simulink model "psm_mpc_bemf_ctrl"  (R2025b)
settings: Solver=ode23tb  StartTime=0.0  StopTime=simlength  FixedStep=tc  MaxStep=tc
values from neighbouring files (symbols this model uses):
  dead_time_INV = 3e-6    (= 3e-06)    [init_model.m]
  emf_fb_p = 0.2    [init_model.m]
  emf_fb_p_ccaller_1 = emf_fb_p    (= 0.2)    [init_model.m]
  emf_fb_p_ccaller_2 = emf_fb_p    (= 0.2)    [init_model.m]
  emf_p = emf_fb_p*4/10    (= 0.08)    [init_model.m]
  emf_p_ccaller_1 = emf_fb_p_ccaller_1*4/10    (= 0.08)    [init_model.m]
  emf_p_ccaller_2 = emf_fb_p_ccaller_2*4/10    (= 0.08)    [init_model.m]
  fPWM_INV = fPWM_AFE    (= 15000)    [init_model.m]
  g0_1Hz = fcut_1Hz_flt * ts_afe * 2*pi    (= 0.000418879020479)    [init_model.m]
  g1_1Hz = 1 - g0_1Hz    (= 0.99958112098)    [init_model.m]
  inv_m_scale = motorc_m_scale    [init_model.m]
  iq_lim = 1.4    [init_model.m]
  k_kalman = 0    [init_model.m]
  kg = Kobs(1)    [init_model.m]
  ki_w = 8    [init_model.m]
  kp_w = 2    [init_model.m]
  kw = Kobs(2)    [init_model.m]
  lim_down_align = -0.2    [init_model.m]
  lim_up_align = 0.2    [init_model.m]
  number_of_modules = 1    [init_model.m]
  omega_m_sim = omega_m_bez    [init_model.m]
  simlength = 2    [init_model.m]
  tc = ts_afe/100    (= 6.66666666667e-07)    [init_model.m]
  time_gain_afe_module_1 = 1.0    (= 1)    [init_model.m]
  time_gain_inv_module_2 = 1.0    (= 1)    [init_model.m]
  time_start_motor_control = 0.035    [init_model.m]
  ts_inv = 1/fPWM_INV    (= 6.66666666667e-05)    [init_model.m]
undefined symbols (not defined in the file or in its folder): ibez, La, Lalpha_norm, Lb, Lbeta_norm, Ls_norm, omega_bez, omega_m_bez, psi_bez, psi_m, psi_m_norm, rpm_base, rpm_bez, Rs, Rs_norm, tau_bez, torque_base, ubez
libraries: fl_lib x24, nesl_utility x11, cstblocks x2, single_phase_pwm_modulator x1, threephase_inductor_lib x1, simple_flexible_shaft x1, psm x1
(part 2 of 2)

== system psm_mpc_bemf_ctrl/inv_psm_mod1/inverter_ctrl1/inverter_control/udc_acquisition ==
  udc_pu : Inport
  Quantizer : Quantizer  QuantizationInterval=adc_quantization
  Unit Delay : UnitDelay  SampleTime=-1  HasFrameUpgradeWarning=on
  Zero-Order Hold : ZeroOrderHold  SampleTime=-1
  udcd_pu : Outport
  wires:
  Quantizer/1 -> Unit Delay/1
  udc_pu/1 -> Zero-Order Hold/1
  Unit Delay/1 -> udcd_pu/1
  Zero-Order Hold/1 -> Quantizer/1

== system psm_mpc_bemf_ctrl/inv_psm_mod1/inverter_ctrl1/inverter_control/encoder-sensorless-switch/double_integrator_observer ==
  theta_psm : Inport
  Dead Zone : DeadZone  LowerValue=-0.01  UpperValue=0.01
  Gain : Gain  Gain=kw
  Gain1 : Gain  Gain=kg
  Gain2 : Gain  Gain=omega_bez
  Gain3 : Gain  Gain=1/omega_bez
  Gain5 : Gain  Gain=ts_inv
  Sum : Sum  Inputs=-+|
  Sum1 : Sum  Inputs=|++
  Sum2 : Sum  Inputs=|++
  Sum8 : Sum  Inputs=++|
  Unit Delay1 : UnitDelay  InitialCondition=pi  SampleTime=-1  HasFrameUpgradeWarning=on
  Unit Delay2 : UnitDelay  SampleTime=-1  HasFrameUpgradeWarning=on
  bounder1 : MATLAB Function  TreatAsAtomicUnit=on
  bounder2 : MATLAB Function  TreatAsAtomicUnit=on
  phase_psm_hat : Outport  VectorParamsAs1DForOutWhenUnconnected=off
  omega_pu_psm_hat : Outport  Port=2  VectorParamsAs1DForOutWhenUnconnected=off
  wires:
  Gain1/1 -> Sum2/1
  theta_psm/1 -> Sum/2
  Sum8/1 -> Unit Delay1/1
  Unit Delay1/1 -> bounder2/1(u)
  Sum1/1 -> Unit Delay2/1
  Gain/1 -> Gain3/1
  Unit Delay2/1 -> omega_pu_psm_hat/1, Sum1/2, Gain5/1
  Sum2/1 -> Sum8/2
  bounder2/1(y) -> Sum2/2, phase_psm_hat/1, Sum/1  "phase_hat"
  bounder1/1(y) -> Gain1/1, Gain/1
  Gain2/1 -> Sum8/1
  Gain3/1 -> Sum1/1
  Gain5/1 -> Gain2/1
  Sum/1 -> bounder1/1(u)

== system psm_mpc_bemf_ctrl/inv_psm_mod1/inverter_ctrl1/inverter_control/inner_ctrl/bemf_observer ==
  ialpha_pu : Inport
  ibeta_pu : Inport  Port=2
  ualpha_pu : Inport  Port=3
  ubeta_pu : Inport  Port=4
  udc_pu : Inport  Port=5
  Mux : Mux  Inputs=3
  Mux1 : Mux  Inputs=3
  Variant Source : VariantSource  VariantControls={use_observer_from_simulink_module_1 == 1, use_observer_from_ccaller_module_1 == 1}
  Variant Source1 : VariantSource  VariantControls={use_observer_from_simulink_module_1 == 1, use_observer_from_ccaller_module_1 == 1}
  bemf observer simulink/ccaller/psm : Scope  NumInputPorts=2
      settings: ActiveDisplayYMinimum=-1.0323324015459419  ActiveDisplayYMaximum=1.1238181835051047
  bemf_observer : Subsystem
  bemf_observer_ccaller : Subsystem
  tag scope: omega_hat_pu_mod1=scoped, phase_hat_mod1=scoped
  wires:
  ialpha_pu/1 -> bemf_observer/1(ialpha_pu), bemf_observer_ccaller/1(ialpha_pu)
  ibeta_pu/1 -> bemf_observer_ccaller/2(ibeta_pu), bemf_observer/2(ibeta_pu)
  Mux/1 -> bemf observer simulink/ccaller/psm/1
  Mux1/1 -> bemf observer simulink/ccaller/psm/2
  ualpha_pu/1 -> bemf_observer_ccaller/3(ualpha_pu), bemf_observer/3(ualpha_pu)
  ubeta_pu/1 -> bemf_observer_ccaller/4(ubeta_pu), bemf_observer/4(ubeta_pu)
  bemf_observer/1(omega_pu) -> Variant Source/1, Mux/1  "omega_pu"
  bemf_observer_ccaller/2(theta_hat) -> Mux1/2, Variant Source1/2  "theta_hat_code"
  bemf_observer_ccaller/1(omega_pu) -> Mux/2, Variant Source/2  "omega_pu_code"
  bemf_observer/2(theta_hat) -> Variant Source1/1, Mux1/1  "theta_hat"
  Variant Source1/1 -> [phase_hat_mod1]
  Variant Source/1 -> [omega_hat_pu_mod1]
  udc_pu/1 -> bemf_observer/5(udc_pu), bemf_observer_ccaller/5(udc_pu)
  [omega_pu_psm] -> Mux/3  "omega_pu_psm"
  [phased_psm] -> Mux1/3  "phased_psm"

== system psm_mpc_bemf_ctrl/inv_psm_mod1/inverter_ctrl1/inverter_control/inner_ctrl/current_reference_generator ==
  torque_ref_pu : Inport
  theta_elec_hat : Inport  Port=2
  Gain5 : Gain  Gain=-1
  Product : Product
  Product1 : Product
  Trigonometric Function1 : Trigonometry
  Trigonometric Function2 : Trigonometry  Operator=cos
  i_alpha_ref : Outport
  i_beta_ref : Outport  Port=2
  tag scope: ialpha_pu_ref_mod1=scoped, ibeta_pu_ref_mod1=scoped
  wires:
  Trigonometric Function1/1 -> Product/2
  Product1/1 -> [ibeta_pu_ref_mod1], i_beta_ref/1
  Trigonometric Function2/1 -> Product1/2
  Product/1 -> Gain5/1
  Gain5/1 -> [ialpha_pu_ref_mod1], i_alpha_ref/1
  torque_ref_pu/1 -> Product/1, Product1/1
  theta_elec_hat/1 -> Trigonometric Function1/1, Trigonometric Function2/1  "theta_electrical"

== system psm_mpc_bemf_ctrl/inv_psm_mod1/inverter_ctrl1/inverter_control/inner_ctrl/current_transformation ==
  Demux : Demux  Outputs=3
  alphabeta2dq : MATLAB Function  TreatAsAtomicUnit=on
  uvw2alphabeta : MATLAB Function  TreatAsAtomicUnit=on
  tag scope: ialpha_pu_mod1=scoped, ibeta_pu_mod1=scoped, id_pu_mod1=scoped, iq_pu_mod1=scoped
  wires:
  alphabeta2dq/2(q) -> [iq_pu_mod1]  "iq_pu"
  alphabeta2dq/1(d) -> [id_pu_mod1]  "id_pu"
  uvw2alphabeta/2(beta) -> alphabeta2dq/2(beta), [ibeta_pu_mod1]  "ibeta_pu"
  uvw2alphabeta/1(alpha) -> [ialpha_pu_mod1], alphabeta2dq/1(alpha)  "ialpha_pu"
  [motor_phase_ctrl_mod1] -> alphabeta2dq/3(gamma)
  Demux/3 -> uvw2alphabeta/3(w)  "iw"
  Demux/2 -> uvw2alphabeta/2(v)  "iv"
  Demux/1 -> uvw2alphabeta/1(u)  "iu"
  [isd_uvw_inv_mod1] -> Demux/1

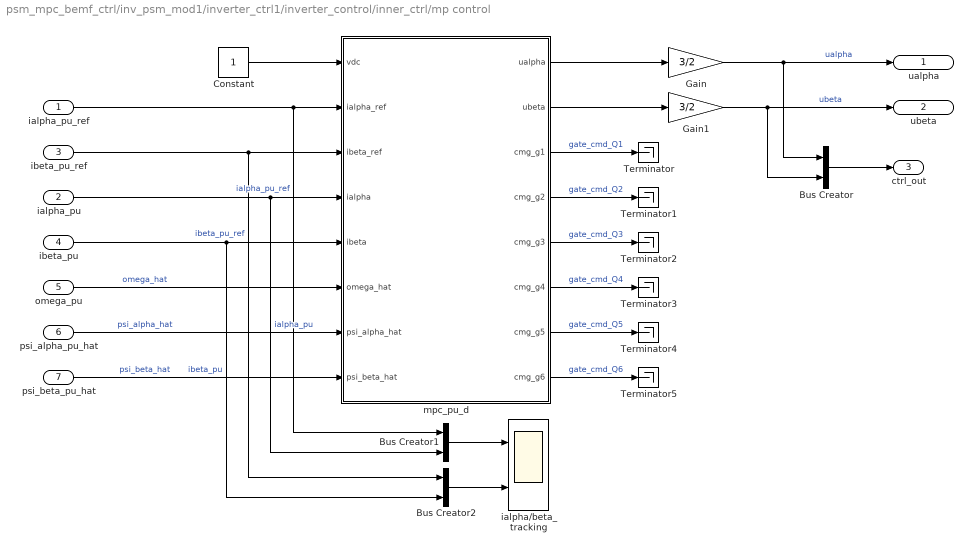
== system psm_mpc_bemf_ctrl/inv_psm_mod1/inverter_ctrl1/inverter_control/inner_ctrl/mp control ==
  ialpha_pu_ref : Inport
  ialpha_pu : Inport  Port=2
  ibeta_pu_ref : Inport  Port=3
  ibeta_pu : Inport  Port=4
  omega_pu : Inport  Port=5
  psi_alpha_pu_hat : Inport  Port=6
  psi_beta_pu_hat : Inport  Port=7
  Bus Creator : BusCreator  Inputs=2
  Bus Creator1 : BusCreator  Inputs=2
  Bus Creator2 : BusCreator  Inputs=2
  Constant : Constant
  Gain : Gain  Gain=3/2
  Gain1 : Gain  Gain=3/2
  Terminator{,1..5} (6 alike) : Terminator
  ialpha/beta_tracking : Scope  NumInputPorts=2
      settings: ActiveDisplayYMinimum=-1.5381312962458753  ActiveDisplayYMaximum=1.5265169032865786  DataLoggingVariableName=ScopeData2
  mpc_pu_d : MATLAB Function  TreatAsAtomicUnit=on
  ualpha : Outport
  ubeta : Outport  Port=2
  ctrl_out : Outport  Port=3
  wires:
  ialpha_pu_ref/1 -> mpc_pu_d/2(ialpha_ref), Bus Creator1/1  "ialpha_pu_ref"
  ibeta_pu_ref/1 -> mpc_pu_d/3(ibeta_ref), Bus Creator2/1  "ibeta_pu_ref"
  ialpha_pu/1 -> mpc_pu_d/4(ialpha), Bus Creator1/2  "ialpha_pu"
  ibeta_pu/1 -> mpc_pu_d/5(ibeta), Bus Creator2/2  "ibeta_pu"
  omega_pu/1 -> mpc_pu_d/6(omega_hat)  "omega_hat"
  psi_alpha_pu_hat/1 -> mpc_pu_d/7(psi_alpha_hat)  "psi_alpha_hat"
  psi_beta_pu_hat/1 -> mpc_pu_d/8(psi_beta_hat)  "psi_beta_hat"
  Constant/1 -> mpc_pu_d/1(vdc)
  Bus Creator1/1 -> ialpha/beta_tracking/1
  Bus Creator2/1 -> ialpha/beta_tracking/2
  Bus Creator/1 -> ctrl_out/1
  mpc_pu_d/1(ualpha) -> Gain/1
  mpc_pu_d/2(ubeta) -> Gain1/1
  mpc_pu_d/3(cmg_g1) -> Terminator/1  "gate_cmd_Q1"
  mpc_pu_d/4(cmg_g2) -> Terminator1/1  "gate_cmd_Q2"
  mpc_pu_d/5(cmg_g3) -> Terminator2/1  "gate_cmd_Q3"
  mpc_pu_d/6(cmg_g4) -> Terminator3/1  "gate_cmd_Q4"
  mpc_pu_d/7(cmg_g5) -> Terminator4/1  "gate_cmd_Q5"
  mpc_pu_d/8(cmg_g6) -> Terminator5/1  "gate_cmd_Q6"
  Gain/1 -> Bus Creator/1, ualpha/1  "ualpha"
  Gain1/1 -> Bus Creator/2, ubeta/1  "ubeta"

== system psm_mpc_bemf_ctrl/inv_psm_mod1/inverter_ctrl1/inverter_control/is inv quantizzation and one step delay/is inv quantizzation and one step delay ==
  is_u_pu : Inport
  is_v_pu : Inport  Port=2
  is_w_pu : Inport  Port=3
  Gain3 : Gain  Gain=-1
  Gain4 : Gain  Gain=-1
  Gain5 : Gain  Gain=-1
  Quantizer : Quantizer  QuantizationInterval=adc_quantization
  Quantizer1 : Quantizer  QuantizationInterval=adc_quantization
  Quantizer2 : Quantizer  QuantizationInterval=adc_quantization
  Unit Delay : UnitDelay  SampleTime=-1  HasFrameUpgradeWarning=on
  Unit Delay1 : UnitDelay  SampleTime=-1  HasFrameUpgradeWarning=on
  Unit Delay2 : UnitDelay  SampleTime=-1  HasFrameUpgradeWarning=on
  Zero-Order Hold : ZeroOrderHold  SampleTime=-1
  Zero-Order Hold1 : ZeroOrderHold  SampleTime=-1
  Zero-Order Hold2 : ZeroOrderHold  SampleTime=-1
  isd_u_pu : Outport
  isd_v_pu : Outport  Port=2
  isd_w_pu : Outport  Port=3
  wires:
  Unit Delay/1 -> Gain3/1
  Unit Delay1/1 -> Gain4/1
  Unit Delay2/1 -> Gain5/1
  Quantizer/1 -> Unit Delay/1
  Quantizer1/1 -> Unit Delay1/1
  Quantizer2/1 -> Unit Delay2/1
  is_u_pu/1 -> Zero-Order Hold/1
  is_v_pu/1 -> Zero-Order Hold1/1
  is_w_pu/1 -> Zero-Order Hold2/1
  Gain3/1 -> isd_u_pu/1
  Gain4/1 -> isd_v_pu/1
  Gain5/1 -> isd_w_pu/1
  Zero-Order Hold/1 -> Quantizer/1
  Zero-Order Hold1/1 -> Quantizer1/1
  Zero-Order Hold2/1 -> Quantizer2/1

== system psm_mpc_bemf_ctrl/inv_psm_mod1/inverter_ctrl1/inverter_control/omega_pu/flt ==
  input : Inport
  Gain3 : Gain  Gain=g1_1Hz
  Gain6 : Gain  Gain=g0_1Hz
  Sum : Sum  Inputs=|++
  Unit Delay1 : UnitDelay  SampleTime=-1  HasFrameUpgradeWarning=on
  output : Outport  VectorParamsAs1DForOutWhenUnconnected=off
  wires:
  Gain6/1 -> Sum/1
  input/1 -> Gain6/1
  Unit Delay1/1 -> Gain3/1
  Gain3/1 -> Sum/2
  Sum/1 -> Unit Delay1/1, output/1

== system psm_mpc_bemf_ctrl/inv_psm_mod1/inverter_ctrl1/inverter_control/phase_compensation_1/alignment_ctrl ==
  local_time : Inport
  master_time : Inport  Port=2
  Constant : Constant  Value=0
  Gain : Gain  Gain=-1
  Sum : Sum  Inputs=|+-
  pi : Subsystem  mask{kp=0 %kp_align, ki=0 %ki_align, lim_up=lim_up_align, lim_down=lim_down_align}
      mask prompts: ki "ki*ts"
      mask Display:
      | disp('pi()');
      | port_label('input', 1, 'u_ref');
      | port_label('input', 2, 'u');
      | port_label('output', 1, 'y');
  dp : Outport
  wires:
  master_time/1 -> Sum/1
  Sum/1 -> Gain/1
  Constant/1 -> pi/1(u_ref)
  local_time/1 -> Sum/2
  Gain/1 -> pi/2(u)
  pi/1(y) -> dp/1

== system psm_mpc_bemf_ctrl/inv_psm_mod1/inverter_ctrl1/inverter_control/speed_reference_generator/flt ==
  input : Inport
  Gain3 : Gain  Gain=g1_1Hz
  Gain6 : Gain  Gain=g0_1Hz
  Sum : Sum  Inputs=|++
  Unit Delay1 : UnitDelay  SampleTime=-1  HasFrameUpgradeWarning=on
  output : Outport  VectorParamsAs1DForOutWhenUnconnected=off
  wires:
  Gain6/1 -> Sum/1
  input/1 -> Gain6/1
  Unit Delay1/1 -> Gain3/1
  Gain3/1 -> Sum/2
  Sum/1 -> Unit Delay1/1, output/1

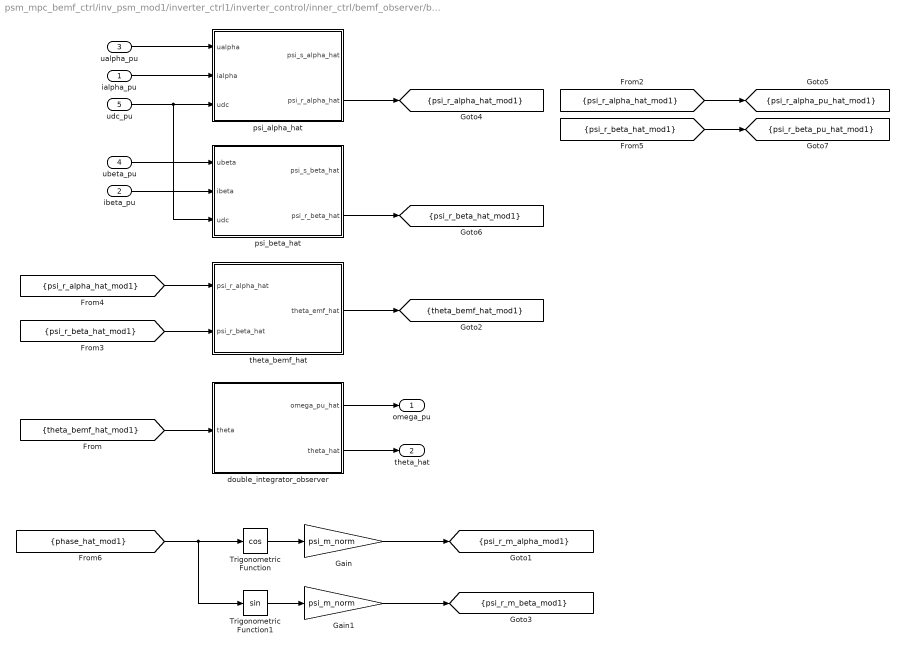
== system psm_mpc_bemf_ctrl/inv_psm_mod1/inverter_ctrl1/inverter_control/inner_ctrl/bemf_observer/bemf_observer ==
  ialpha_pu : Inport
  ibeta_pu : Inport  Port=2
  ualpha_pu : Inport  Port=3
  ubeta_pu : Inport  Port=4
  udc_pu : Inport  Port=5
  Gain : Gain  Gain=psi_m_norm
  Gain1 : Gain  Gain=psi_m_norm
  Trigonometric Function : Trigonometry  Operator=cos
  Trigonometric Function1 : Trigonometry
  double_integrator_observer : Subsystem
  psi_alpha_hat : Subsystem
  psi_beta_hat : Subsystem
  theta_bemf_hat : Subsystem
  omega_pu : Outport
  theta_hat : Outport  Port=2
  tag scope: psi_r_alpha_hat_mod1=scoped, psi_r_alpha_pu_hat_mod1=scoped, psi_r_beta_hat_mod1=scoped, psi_r_beta_pu_hat_mod1=scoped, psi_r_m_alpha_mod1=scoped, psi_r_m_beta_mod1=scoped, theta_bemf_hat_mod1=scoped
  wires:
  Trigonometric Function/1 -> Gain/1
  Trigonometric Function1/1 -> Gain1/1
  ialpha_pu/1 -> psi_alpha_hat/2(ialpha)
  ibeta_pu/1 -> psi_beta_hat/2(ibeta)
  psi_alpha_hat/2(psi_r_alpha_hat) -> [psi_r_alpha_hat_mod1]
  psi_beta_hat/2(psi_r_beta_hat) -> [psi_r_beta_hat_mod1]
  [psi_r_alpha_hat_mod1] -> theta_bemf_hat/1(psi_r_alpha_hat)
  [psi_r_beta_hat_mod1] -> theta_bemf_hat/2(psi_r_beta_hat)
  ualpha_pu/1 -> psi_alpha_hat/1(ualpha)
  ubeta_pu/1 -> psi_beta_hat/1(ubeta)
  [phase_hat_mod1] -> Trigonometric Function/1, Trigonometric Function1/1
  Gain/1 -> [psi_r_m_alpha_mod1]
  Gain1/1 -> [psi_r_m_beta_mod1]
  theta_bemf_hat/1(theta_emf_hat) -> [theta_bemf_hat_mod1]
  [theta_bemf_hat_mod1] -> double_integrator_observer/1(theta)
  double_integrator_observer/1(omega_pu_hat) -> omega_pu/1
  double_integrator_observer/2(theta_hat) -> theta_hat/1
  [psi_r_alpha_hat_mod1] -> [psi_r_alpha_pu_hat_mod1]
  [psi_r_beta_hat_mod1] -> [psi_r_beta_pu_hat_mod1]
  udc_pu/1 -> psi_beta_hat/3(udc), psi_alpha_hat/3(udc)

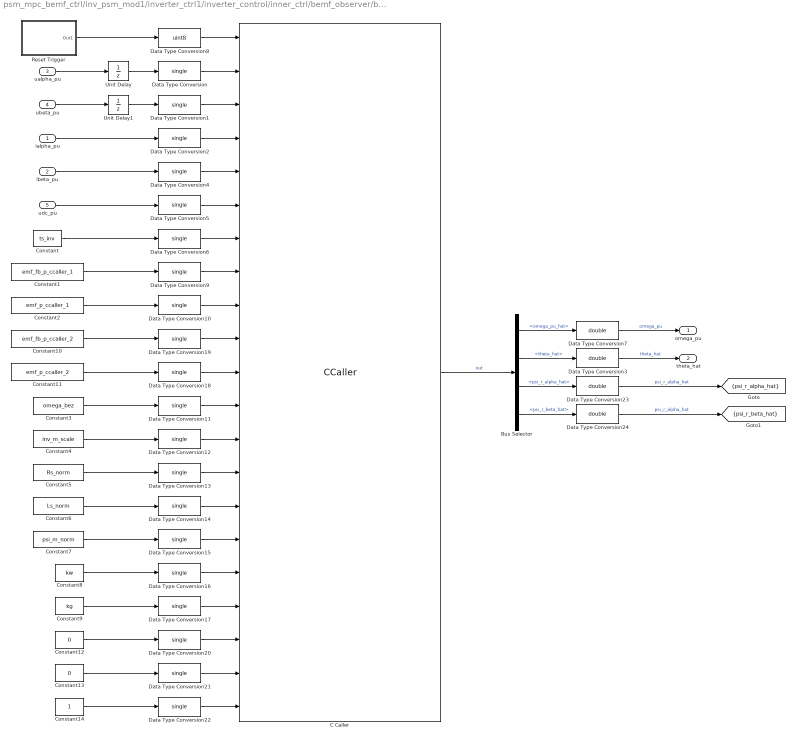
== system psm_mpc_bemf_ctrl/inv_psm_mod1/inverter_ctrl1/inverter_control/inner_ctrl/bemf_observer/bemf_observer_ccaller ==
  ialpha_pu : Inport
  ibeta_pu : Inport  Port=2
  ualpha_pu : Inport  Port=3
  ubeta_pu : Inport  Port=4
  udc_pu : Inport  Port=5
  Bus Selector : BusSelector  OutputSignals=omega_pu_hat,theta_hat,psi_r_alpha_hat,psi_r_beta_hat
  C Caller : CCaller  FunctionName=bemf_obsv_process_simulink  PortSpecificationStruct="%)30     .    N\"8   8    (     @         %    \"    !8    !     0         %  0 \"0    $    _    07)G3F%M90  4&]R=$YA;64 4V-O<&4     26YD97@     5'EP90      4VEZ90      27-';&]B86P   X    P    !@    @    $          4    (     0    ,    !         !   P!O=70 #@   #     &    \"     0         !0    @    !     P    $         $  # &]U=  .    .     8    (    !          %    \"     $    &     0         0  ...(+12985 chars)"
  Constant : Constant  Value=ts_inv
  Constant1 : Constant  Value=emf_fb_p_ccaller_1
  Constant10 : Constant  Value=emf_fb_p_ccaller_2
  Constant11 : Constant  Value=emf_p_ccaller_2
  Constant12 : Constant  Value=0
  Constant13 : Constant  Value=0
  Constant14 : Constant
  Constant2 : Constant  Value=emf_p_ccaller_1
  Constant3 : Constant  Value=omega_bez
  Constant4 : Constant  Value=inv_m_scale
  Constant5 : Constant  Value=Rs_norm
  Constant6 : Constant  Value=Ls_norm
  Constant7 : Constant  Value=psi_m_norm
  Constant8 : Constant  Value=kw
  Constant9 : Constant  Value=kg
  Data Type Conversion{,1..2,4..6,9..22} (20 alike) : DataTypeConversion  OutDataTypeStr=single  SaturateOnIntegerOverflow=off  RndMeth=Floor
  Data Type Conversion{3,7,23..24} (4 alike) : DataTypeConversion  OutDataTypeStr=double  SaturateOnIntegerOverflow=off  RndMeth=Floor
  Data Type Conversion8 : DataTypeConversion  OutDataTypeStr=uint8  SaturateOnIntegerOverflow=off  RndMeth=Floor
  Reset Trigger : Subsystem
  Unit Delay : UnitDelay  SampleTime=-1  HasFrameUpgradeWarning=on
  Unit Delay1 : UnitDelay  SampleTime=-1  HasFrameUpgradeWarning=on
  omega_pu : Outport
  theta_hat : Outport  Port=2
  tag scope: psi_r_alpha_hat=scoped, psi_r_beta_hat=scoped
  wires:
  Data Type Conversion5/1 -> C Caller/6
  Data Type Conversion/1 -> C Caller/2
  C Caller/1 -> Bus Selector/1  "out"
  Data Type Conversion1/1 -> C Caller/3
  Data Type Conversion4/1 -> C Caller/5
  Data Type Conversion2/1 -> C Caller/4
  Data Type Conversion6/1 -> C Caller/7
  Bus Selector/2 -> Data Type Conversion3/1  "<theta_hat>"
  Bus Selector/1 -> Data Type Conversion7/1  "<omega_pu_hat>"
  Data Type Conversion7/1 -> omega_pu/1  "omega_pu"
  Data Type Conversion3/1 -> theta_hat/1  "theta_hat"
  Data Type Conversion8/1 -> C Caller/1
  Data Type Conversion9/1 -> C Caller/8
  Data Type Conversion10/1 -> C Caller/9
  Data Type Conversion19/1 -> C Caller/10
  Data Type Conversion18/1 -> C Caller/11
  Data Type Conversion11/1 -> C Caller/12
  Data Type Conversion12/1 -> C Caller/13
  Data Type Conversion13/1 -> C Caller/14
  Data Type Conversion14/1 -> C Caller/15
  Data Type Conversion15/1 -> C Caller/16
  Data Type Conversion16/1 -> C Caller/17
  Data Type Conversion17/1 -> C Caller/18
  Data Type Conversion20/1 -> C Caller/19
  Data Type Conversion21/1 -> C Caller/20
  Data Type Conversion22/1 -> C Caller/21
  Constant14/1 -> Data Type Conversion22/1
  Constant13/1 -> Data Type Conversion21/1
  Constant12/1 -> Data Type Conversion20/1
  Constant9/1 -> Data Type Conversion17/1
  Constant8/1 -> Data Type Conversion16/1
  Constant7/1 -> Data Type Conversion15/1
  Constant6/1 -> Data Type Conversion14/1
  Constant5/1 -> Data Type Conversion13/1
  Constant4/1 -> Data Type Conversion12/1
  Constant3/1 -> Data Type Conversion11/1
  Constant11/1 -> Data Type Conversion18/1
  Constant10/1 -> Data Type Conversion19/1
  Constant2/1 -> Data Type Conversion10/1
  Constant1/1 -> Data Type Conversion9/1
  Constant/1 -> Data Type Conversion6/1
  ibeta_pu/1 -> Data Type Conversion4/1
  ialpha_pu/1 -> Data Type Conversion2/1
  ubeta_pu/1 -> Unit Delay1/1
  ualpha_pu/1 -> Unit Delay/1
  Reset Trigger/1(Out1) -> Data Type Conversion8/1
  udc_pu/1 -> Data Type Conversion5/1
  Bus Selector/3 -> Data Type Conversion23/1  "<psi_r_alpha_hat>"
  Data Type Conversion23/1 -> [psi_r_alpha_hat]  "psi_r_alpha_hat"
  Data Type Conversion24/1 -> [psi_r_beta_hat]  "psi_r_alpha_hat"
  Bus Selector/4 -> Data Type Conversion24/1  "<psi_r_beta_hat>"
  Unit Delay/1 -> Data Type Conversion/1
  Unit Delay1/1 -> Data Type Conversion1/1

== system psm_mpc_bemf_ctrl/inv_psm_mod1/inverter_ctrl1/inverter_control/phase_compensation_1/alignment_ctrl/pi ==
  u_ref : Inport
  u : Inport  Port=2
  1/Ti : Gain  Gain=kp  SaturateOnIntegerOverflow=on  OutDataTypeStr=Inherit: Same as input  ParamDataTypeStr=Inherit: Same as input
  Saturation : Saturate  UpperLimit=lim_up  LowerLimit=lim_down
  Sum1 : Sum  Inputs=+++  SaturateOnIntegerOverflow=on
  Sum2 : Sum  Inputs=-+  SaturateOnIntegerOverflow=on
  Sum3 : Sum  Inputs=-+  SaturateOnIntegerOverflow=on
  Unit Delay4 : UnitDelay  SampleTime=-1  HasFrameUpgradeWarning=on
  kp : Gain  Gain=ki  SaturateOnIntegerOverflow=on  OutDataTypeStr=Inherit: Same as input  ParamDataTypeStr=Inherit: Same as input
  y : Outport
  wires:
  1/Ti/1 -> Sum1/1, Sum3/1
  kp/1 -> Sum1/2
  Sum3/1 -> Unit Delay4/1
  Unit Delay4/1 -> Sum1/3
  u_ref/1 -> Sum2/2
  u/1 -> Sum2/1
  Sum2/1 -> kp/1, 1/Ti/1
  Sum1/1 -> Saturation/1
  Saturation/1 -> Sum3/2, y/1

== system psm_mpc_bemf_ctrl/inv_psm_mod1/inverter_ctrl1/inverter_control/inner_ctrl/bemf_observer/bemf_observer/double_integrator_observer ==
  theta : Inport
  Dead Zone : DeadZone  LowerValue=-0.01  UpperValue=0.01
  Gain : Gain  Gain=kw
  Gain1 : Gain  Gain=kg
  Gain2 : Gain  Gain=omega_bez
  Gain3 : Gain  Gain=1/omega_bez
  Gain5 : Gain  Gain=ts_inv
  Sum : Sum  Inputs=-+|
  Sum1 : Sum  Inputs=|++
  Sum2 : Sum  Inputs=|++
  Sum8 : Sum  Inputs=++|
  Unit Delay1 : UnitDelay  InitialCondition=pi  SampleTime=-1  HasFrameUpgradeWarning=on
  Unit Delay2 : UnitDelay  SampleTime=-1  HasFrameUpgradeWarning=on
  bounder1 : MATLAB Function  TreatAsAtomicUnit=on
  bounder2 : MATLAB Function  TreatAsAtomicUnit=on
  omega_pu_hat : Outport  VectorParamsAs1DForOutWhenUnconnected=off
  theta_hat : Outport  Port=2  VectorParamsAs1DForOutWhenUnconnected=off
  wires:
  Gain1/1 -> Sum2/1
  theta/1 -> Sum/2  "theta_bemf"
  Sum8/1 -> Unit Delay1/1
  Unit Delay1/1 -> bounder2/1(u)
  Sum1/1 -> Unit Delay2/1
  Gain/1 -> Gain3/1
  Unit Delay2/1 -> omega_pu_hat/1, Sum1/2, Gain5/1
  Sum2/1 -> Sum8/2
  bounder2/1(y) -> Sum2/2, theta_hat/1, Sum/1  "theta_hat"
  bounder1/1(y) -> Gain1/1, Gain/1
  Gain2/1 -> Sum8/1
  Gain3/1 -> Sum1/1
  Gain5/1 -> Gain2/1
  Sum/1 -> bounder1/1(u)

== system psm_mpc_bemf_ctrl/inv_psm_mod1/inverter_ctrl1/inverter_control/inner_ctrl/bemf_observer/bemf_observer/psi_alpha_hat ==
  ualpha : Inport
  ialpha : Inport  Port=2
  udc : Inport  Port=3
  Gain1 : Gain  Gain=Rs_norm
  Gain2 : Gain  Gain=emf_fb_p
  Gain3 : Gain  Gain=emf_p
  Gain4 : Gain  Gain=omega_bez
  Gain5 : Gain  Gain=Ls_norm
  Gain6 : Gain  Gain=inv_m_scale
  Gain7 : Gain  Gain=ts_inv
  Product : Product  RndMeth=Zero
  Sum : Sum  Inputs=|+-
  Sum1 : Sum  Inputs=|+-
  Sum2 : Sum  Inputs=++-  SaturateOnIntegerOverflow=on
  Sum3 : Sum  Inputs=|++
  Sum4 : Sum  Inputs=+-  SaturateOnIntegerOverflow=on
  Unit Delay1 : UnitDelay  SampleTime=-1  HasFrameUpgradeWarning=on
  Unit Delay3 : UnitDelay  SampleTime=-1  HasFrameUpgradeWarning=on
  psi_s_alpha_hat : Outport  VectorParamsAs1DForOutWhenUnconnected=off
  psi_r_alpha_hat : Outport  Port=2  VectorParamsAs1DForOutWhenUnconnected=off
  wires:
  [psi_r_m_alpha_mod1] -> Sum1/1
  [psi_r_alpha_hat_mod1] -> Sum1/2
  Gain4/1 -> Gain7/1
  Sum2/1 -> Gain4/1
  Gain3/1 -> Sum2/3
  ialpha/1 -> Gain5/1, Gain1/1
  Gain1/1 -> Sum/2
  Sum/1 -> Sum2/2
  ualpha/1 -> Product/1
  Gain5/1 -> Unit Delay3/1
  Unit Delay1/1 -> Sum4/1, psi_s_alpha_hat/1, Gain3/1, Sum3/2
  Sum3/1 -> Unit Delay1/1
  Sum1/1 -> Gain2/1
  Gain2/1 -> Sum2/1
  Gain7/1 -> Sum3/1
  Product/1 -> Gain6/1
  Gain6/1 -> Sum/1
  Sum4/1 -> psi_r_alpha_hat/1
  Unit Delay3/1 -> Sum4/2
  udc/1 -> Product/2

== system psm_mpc_bemf_ctrl/inv_psm_mod1/inverter_ctrl1/inverter_control/inner_ctrl/bemf_observer/bemf_observer/psi_beta_hat ==
  ubeta : Inport
  ibeta : Inport  Port=2
  udc : Inport  Port=3
  Gain1 : Gain  Gain=Rs_norm
  Gain2 : Gain  Gain=emf_fb_p
  Gain3 : Gain  Gain=emf_p
  Gain4 : Gain  Gain=omega_bez
  Gain5 : Gain  Gain=Ls_norm
  Gain6 : Gain  Gain=inv_m_scale
  Gain7 : Gain  Gain=ts_inv
  Product : Product  RndMeth=Zero
  Sum : Sum  Inputs=|+-
  Sum1 : Sum  Inputs=|+-
  Sum2 : Sum  Inputs=++-  SaturateOnIntegerOverflow=on
  Sum3 : Sum  Inputs=|++
  Sum4 : Sum  Inputs=+-  SaturateOnIntegerOverflow=on
  Unit Delay1 : UnitDelay  SampleTime=-1  HasFrameUpgradeWarning=on
  Unit Delay3 : UnitDelay  SampleTime=-1  HasFrameUpgradeWarning=on
  psi_s_beta_hat : Outport  VectorParamsAs1DForOutWhenUnconnected=off
  psi_r_beta_hat : Outport  Port=2  VectorParamsAs1DForOutWhenUnconnected=off
  wires:
  Gain5/1 -> Unit Delay3/1
  Sum/1 -> Sum2/2
  Gain1/1 -> Sum/2
  ibeta/1 -> Gain5/1, Gain1/1
  Gain3/1 -> Sum2/3
  Sum2/1 -> Gain4/1
  Gain4/1 -> Gain7/1
  Sum1/1 -> Gain2/1
  [psi_r_beta_hat_mod1] -> Sum1/2
  [psi_r_m_beta_mod1] -> Sum1/1
  Unit Delay1/1 -> Gain3/1, Sum4/1, psi_s_beta_hat/1, Sum3/2
  Sum3/1 -> Unit Delay1/1
  Gain2/1 -> Sum2/1
  ubeta/1 -> Product/1
  Gain7/1 -> Sum3/1
  Product/1 -> Gain6/1
  Gain6/1 -> Sum/1
  Sum4/1 -> psi_r_beta_hat/1
  Unit Delay3/1 -> Sum4/2
  udc/1 -> Product/2

== system psm_mpc_bemf_ctrl/inv_psm_mod1/inverter_ctrl1/inverter_control/inner_ctrl/bemf_observer/bemf_observer/theta_bemf_hat ==
  psi_r_alpha_hat : Inport
  psi_r_beta_hat : Inport  Port=2
  Trigonometric Function : Trigonometry  Operator=atan2  OutputSignalType=real
  theta_emf_hat : Outport  VectorParamsAs1DForOutWhenUnconnected=off
  wires:
  psi_r_alpha_hat/1 -> Trigonometric Function/2
  psi_r_beta_hat/1 -> Trigonometric Function/1
  Trigonometric Function/1 -> theta_emf_hat/1

== system psm_mpc_bemf_ctrl/inv_psm_mod1/inverter_ctrl1/inverter_control/inner_ctrl/bemf_observer/bemf_observer_ccaller/Reset Trigger ==
  Step : Step  Time=0.01  Before=1  After=0
  Out1 : Outport
  wires:
  Step/1 -> Out1/1  "Reset"

== matlab function psm_mpc_bemf_ctrl/inv_psm_mod1/inverter_ctrl1/inverter_control/inner_ctrl/mp control/mpc_pu_d ==
  data: vdc input; ialpha_ref input; ibeta_ref input; ialpha input; ualpha output; ibeta input; omega_hat input; psi_alpha_hat input; psi_beta_hat input; ubeta output; cmg_g1 output; cmg_g2 output; cmg_g3 output; cmg_g4 output; cmg_g5 output; cmg_g6 output; Rs_norm parameter; Lalpha_norm parameter; Lbeta_norm parameter; ts_inv parameter; k_kalman parameter; omega_bez parameter
function [ualpha, ubeta, cmg_g1, cmg_g2, cmg_g3, cmg_g4, cmg_g5, cmg_g6]    = mpc(vdc, ialpha_ref,...
    ibeta_ref, ialpha, ibeta, omega_hat, psi_alpha_hat, psi_beta_hat, Rs_norm, Lalpha_norm, Lbeta_norm, ...
    ts_inv, k_kalman, omega_bez)

    persistent ualpha_z ubeta_z

    on = 15;
    off = 0;

    ualpha_1 = 2/3*vdc;
    ubeta_1 = 0;

    ualpha_2 = 2/3*1/2*vdc;
    ubeta_2 = 2/3*sqrt(3)/2*vdc;

    ualpha_3 = -2/3*1/2*vdc;
    ubeta_3 = 2/3*sqrt(3)/2*vdc;

    ualpha_4 = -2/3*vdc;
    ubeta_4 = 0;

    ualpha_5 = -2/3*1/2*vdc;
    ubeta_5 = -2/3*sqrt(3)/2*vdc;

    ualpha_6 = 2/3*1/2*vdc;
    ubeta_6 = -2/3*sqrt(3)/2*vdc;

    ualpha_0 = 0;
    ubeta_0 = 0;

    if isempty(ualpha_z)
        ualpha_z = 0;
        ubeta_z = 0;
    end
    ts = ts_inv*omega_bez;

    ia_p0 = (1-Rs_norm/Lalpha_norm*ts)*ialpha + omega_hat/Lalpha_norm*psi_beta_hat*ts + ualpha_0*ts/Lalpha_norm;
    ib_p0 = (1-Rs_norm/Lbeta_norm*ts)*ibeta - omega_hat/Lbeta_norm*psi_alpha_hat*ts + ubeta_0*ts/Lbeta_norm;
    
    ia_p1 = (1-Rs_norm/Lalpha_norm*ts)*ialpha + omega_hat/Lalpha_norm*psi_beta_hat*ts + ualpha_1*ts/Lalpha_norm;
    ib_p1 = (1-Rs_norm/Lbeta_norm*ts)*ibeta - omega_hat/Lbeta_norm*psi_alpha_hat*ts + ubeta_1*ts/Lbeta_norm;

    ia_p2 = (1-Rs_norm/Lalpha_norm*ts)*ialpha + omega_hat/Lalpha_norm*psi_beta_hat*ts + ualpha_2*ts/Lalpha_norm;
    ib_p2 = (1-Rs_norm/Lbeta_norm*ts)*ibeta - omega_hat/Lbeta_norm*psi_alpha_hat*ts + ubeta_2*ts/Lbeta_norm;

    ia_p3 = (1-Rs_norm/Lalpha_norm*ts)*ialpha + omega_hat/Lalpha_norm*psi_beta_hat*ts + ualpha_3*ts/Lalpha_norm;
    ib_p3 = (1-Rs_norm/Lbeta_norm*ts)*ibeta - omega_hat/Lbeta_norm*psi_alpha_hat*ts + ubeta_3*ts/Lbeta_norm;

    ia_p4 = (1-Rs_norm/Lalpha_norm*ts)*ialpha + omega_hat/Lalpha_norm*psi_beta_hat*ts + ualpha_4*ts/Lalpha_norm;
    ib_p4 = (1-Rs_norm/Lbeta_norm*ts)*ibeta - omega_hat/Lbeta_norm*psi_alpha_hat*ts + ubeta_4*ts/Lbeta_norm;

    ia_p5 = (1-Rs_norm/Lalpha_norm*ts)*ialpha + omega_hat/Lalpha_norm*psi_beta_hat*ts + ualpha_5*ts/Lalpha_norm;
    ib_p5 = (1-Rs_norm/Lbeta_norm*ts)*ibeta - omega_hat/Lbeta_norm*psi_alpha_hat*ts + ubeta_5*ts/Lbeta_norm;

    ia_p6 = (1-Rs_norm/Lalpha_norm*ts)*ialpha + omega_hat/Lalpha_norm*psi_beta_hat*ts + ualpha_6*ts/Lalpha_norm;
    ib_p6 = (1-Rs_norm/Lbeta_norm*ts)*ibeta - omega_hat/Lbeta_norm*psi_alpha_hat*ts + ubeta_6*ts/Lbeta_norm;
  
    J0 = (ialpha_ref - ia_p0)^2 + (ibeta_ref - ib_p0)^2 + k_kalman * (ualpha_0^2 + ubeta_0^2);
    J1 = (ialpha_ref - ia_p1)^2 + (ibeta_ref - ib_p1)^2 + k_kalman * (ualpha_1^2 + ubeta_1^2);
    J2 = (ialpha_ref - ia_p2)^2 + (ibeta_ref - ib_p2)^2 + k_kalman * (ualpha_2^2 + ubeta_2^2);
    J3 = (ialpha_ref - ia_p3)^2 + (ibeta_ref - ib_p3)^2 + k_kalman * (ualpha_3^2 + ubeta_3^2);
    J4 = (ialpha_ref - ia_p4)^2 + (ibeta_ref - ib_p4)^2 + k_kalman * (ualpha_4^2 + ubeta_4^2);
    J5 = (ialpha_ref - ia_p5)^2 + (ibeta_ref - ib_p5)^2 + k_kalman * (ualpha_5^2 + ubeta_5^2);
    J6 = (ialpha_ref - ia_p6)^2 + (ibeta_ref - ib_p6)^2 + k_kalman * (ualpha_6^2 + ubeta_6^2);
    
    if (ualpha_z == ualpha_0) && (ubeta_z == ubeta_0)
        [m,i] = min([J0, J1, J2, J3, J4, J5, J6]);
        if i == 1
            ualpha = ualpha_0;
            ubeta = ubeta_0;
        elseif i == 2
            ualpha = ualpha_1;
            ubeta = ubeta_1;
        elseif i == 3
            ualpha = ualpha_2;
            ubeta = ubeta_2;
        elseif i == 4
            ualpha = ualpha_3;
            ubeta = ubeta_3;
        elseif i == 5
            ualpha = ualpha_4;
            ubeta = ubeta_4;
        elseif i == 6
            ualpha = ualpha_5;
            ubeta = ubeta_5;
        else
            ualpha = ualpha_6;
            ubeta = ubeta_6;
        end
    elseif (ualpha_z == ualpha_1) && (ubeta_z == ubeta_1)
        [m,i] = min([J0, J1, J2, J6]);
        if i == 1
            ualpha = ualpha_0;
            ubeta = ubeta_0;
        elseif i == 2
            ualpha = ualpha_1;
            ubeta = ubeta_1;
        elseif i == 3
            ualpha = ualpha_2;
            ubeta = ubeta_2;
        else
            ualpha = ualpha_6;
            ubeta = ubeta_6;
        end
    elseif (ualpha_z == ualpha_2) && (ubeta_z == ubeta_2) % vector u2
        [m,i] = min([J0, J1, J2, J3]);
        if i == 1
            ualpha = ualpha_0;
            ubeta = ubeta_0;
        elseif i == 2
            ualpha = ualpha_1;
            ubeta = ubeta_1;
        elseif i == 3
            ualpha = ualpha_2;
            ubeta = ubeta_2;
        else
            ualpha = ualpha_3;
            ubeta = ubeta_3;
        end
    elseif (ualpha_z == ualpha_3) && (ubeta_z == ubeta_3)
        [m,i] = min([J0, J2, J3, J4]);
        if i == 1
            ualpha = ualpha_0;
            ubeta = ubeta_0;
        elseif i == 2
            ualpha = ualpha_2;
            ubeta = ubeta_2;
        elseif i == 3
            ualpha = ualpha_3;
            ubeta = ubeta_3;
        else
            ualpha = ualpha_4;
            ubeta = ubeta_4;
        end
    elseif (ualpha_z == ualpha_4) && (ubeta_z == ubeta_4)
        [m,i] = min([J0, J3, J4, J5]);
        if i == 1
            ualpha = ualpha_0;
            ubeta = ubeta_0;
        elseif i == 2
            ualpha = ualpha_3;
            ubeta = ubeta_3;
        elseif i == 3
            ualpha = ualpha_4;
            ubeta = ubeta_4;
        else
            ualpha = ualpha_5;
            ubeta = ubeta_5;
        end
    elseif (ualpha_z == ualpha_5) && (ubeta_z == ubeta_5) % u5
        [m,i] = min([J0, J4, J5, J6]);
        if i == 1
            ualpha = ualpha_0;
            ubeta = ubeta_0;
        elseif i == 2
            ualpha = ualpha_4;
            ubeta = ubeta_4;
        elseif i == 3
            ualpha = ualpha_5;
            ubeta = ubeta_5;
        else
            ualpha = ualpha_6;
            ubeta = ubeta_6;
        end
    else
        [m,i] = min([J0, J5, J6, J1]);
        if i == 1
            ualpha = ualpha_0;
            ubeta = ubeta_0;
        elseif i == 2
            ualpha = ualpha_5;
            ubeta = ubeta_5;
        elseif i == 3
            ualpha = ualpha_6;
            ubeta = ubeta_6;
        else
            ualpha = ualpha_1;
            ubeta = ubeta_1;
        end
    end
    ualpha_z = ualpha;
    ubeta_z = ubeta;

    if (ualpha == ualpha_0 && ubeta == ubeta_0)
        cmg_g1 = on;
        cmg_g2 = off;
        cmg_g3 = on;
        cmg_g4 = off;
        cmg_g5 = on;
        cmg_g6 = off;
    elseif (ualpha == ualpha_1 && ubeta == ubeta_1)
        cmg_g1 = on;
        cmg_g2 = off;
        cmg_g3 = off;
        cmg_g4 = on;
        cmg_g5 = off;
        cmg_g6 = on;
    elseif (ualpha == ualpha_2 && ubeta == ubeta_2)
        cmg_g1 = on;
        cmg_g2 = off;
        cmg_g3 = on;
        cmg_g4 = off;
        cmg_g5 = off;
        cmg_g6 = on;
    elseif (ualpha == ualpha_3 && ubeta == ubeta_3)
        cmg_g1 = off;
        cmg_g2 = on;
        cmg_g3 = on;
        cmg_g4 = off;
        cmg_g5 = off;
        cmg_g6 = on;
    elseif (ualpha == ualpha_4 && ubeta == ubeta_4)
        cmg_g1 = off;
        cmg_g2 = on;
        cmg_g3 = on;
        cmg_g4 = off;
        cmg_g5 = on;
        cmg_g6 = off;
    elseif (ualpha == ualpha_5 && ubeta == ubeta_5)
        cmg_g1 = off;
        cmg_g2 = on;
        cmg_g3 = off;
        cmg_g4 = on;
        cmg_g5 = on;
        cmg_g6 = off;
    elseif (ualpha == ualpha_6 && ubeta == ubeta_6)
        cmg_g1 = on;
        cmg_g2 = off;
        cmg_g3 = off;
        cmg_g4 = on;
        cmg_g5 = on;
        cmg_g6 = off;
    else
        cmg_g1 = off;
        cmg_g2 = on;
        cmg_g3 = off;
        cmg_g4 = on;
        cmg_g5 = off;
        cmg_g6 = on;
    end  
end

== matlab function psm_mpc_bemf_ctrl/inv_psm_mod1/inverter/timer/MATLAB Function ==
  data: t input; y output; phase input; period input
function y = ramp_up_down(t,phase,period)
x = sin(2*pi/period*t - phase -pi/2);
y = asin(x)/pi + 1/2;

== matlab function psm_mpc_bemf_ctrl/inv_psm_mod1/inverter_ctrl1/inverter_control/encoder-sensorless-switch/double_integrator_observer/bounder1 ==
  data: u input; y output
function y = bounder(u)
    y = -pi + mod(u+3*pi,2*pi);
end

== matlab function psm_mpc_bemf_ctrl/inv_psm_mod1/inverter_ctrl1/inverter_control/encoder-sensorless-switch/double_integrator_observer/bounder2 ==
  data: u input; y output
function y = bounder(u)
    y = -pi + mod(u+3*pi,2*pi);
end

== matlab function psm_mpc_bemf_ctrl/inv_psm_mod1/inverter/MATLAB Function ==
  data: ua input; uu output; uv output; uw output; ub input
function [uu, uv, uw] = ab2uvw(ua, ub)

uu = ua;
uv = -ua/2 + sqrt(3)/2*ub;
uw = -ua/2 - sqrt(3)/2*ub;

== matlab function psm_mpc_bemf_ctrl/inv_psm_mod1/inverter_ctrl1/inverter_control/encoder-sensorless-switch/MATLAB Function ==
  data: omega_ctrl output; phase_psm input; omega_obs input; phase_obs input; phase_ctrl output; omega_psm input; omega_th parameter
function [omega_ctrl, phase_ctrl] = switch_enc2obs(phase_psm, omega_obs, phase_obs, omega_psm, omega_th)

if abs(omega_psm) > omega_th
    omega_ctrl = omega_obs;
    phase_ctrl = phase_obs;
else
    omega_ctrl = omega_psm;
    phase_ctrl = phase_psm;
end

== matlab function psm_mpc_bemf_ctrl/inv_psm_mod1/inverter_ctrl1/inverter_control/inner_ctrl/bemf_observer/bemf_observer/double_integrator_observer/bounder1 ==
  data: u input; y output
function y = bounder(u)
    
    y = -pi + mod(u+3*pi,2*pi);
end

== matlab function psm_mpc_bemf_ctrl/inv_psm_mod1/inverter_ctrl1/inverter_control/inner_ctrl/bemf_observer/bemf_observer/double_integrator_observer/bounder2 ==
  data: u input; y output
function y = bounder(u)
    
    u = -pi + mod(u+3*pi,2*pi);
    
    y = u;
end

== matlab function psm_mpc_bemf_ctrl/inv_psm_mod1/inverter_ctrl1/inverter_control/inner_ctrl/current_transformation/alphabeta2dq ==
  data: alpha input; d output; beta input; gamma input; q output
function [d,q] = alphabeta2dq(alpha,beta,gamma)

    d  =  alpha*cos(gamma) + beta*sin(gamma);
    q = -alpha*sin(gamma) + beta*cos(gamma);

end

== matlab function psm_mpc_bemf_ctrl/inv_psm_mod1/inverter_ctrl1/inverter_control/inner_ctrl/current_transformation/uvw2alphabeta ==
  data: u input; alpha output; v input; w input; beta output
function [alpha,beta] = uvw2alphabeta(u,v,w)

alpha = 2/3*(u - 1/2*v - 1/2*w);
beta  = 2/3*(sqrt(3)/2*(v - w));

end
